simulink model "sensor"  (Simulink 4.00)
settings: Solver=ode45  StartTime=0.0  StopTime=0.5  MaxStep=1/80000  RelTol=1e-3
settings Model: LastModifiedBy=Gui

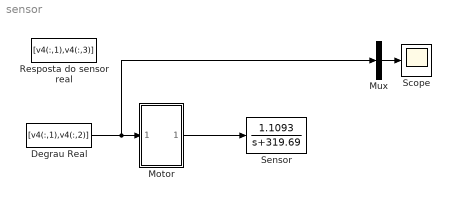
== system sensor ==
  Degrau Real : FromWorkspace  VariableName=[v4(:,1),v4(:,2)]  SampleTime=0  OutputAfterFinalValue=Extrapolation
  Motor : Subsystem
      settings: RTWFcnNameOpts=Auto  RTWFileNameOpts=Auto
  Mux : Mux  Inputs=3
  Resposta do sensor real : FromWorkspace  VariableName=[v4(:,1),v4(:,3)]  SampleTime=0  OutputAfterFinalValue=Extrapolation
  Scope : Scope
      settings: TimeRange=0.5  YMin=0  YMax=10  SaveToWorkspace=off  SaveName=ScopeData  MaxDataPoints=5000
  "Sensor " : TransferFcn  Numerator=1.1093  Denominator=[1 319.69]  AbsoluteTolerance=auto  Realization=auto
  wires:
  Degrau Real/1 -> Motor/1(In1), Mux/2
  Mux/1 -> Scope/1
  Motor/1(Out1) -> "Sensor "/1

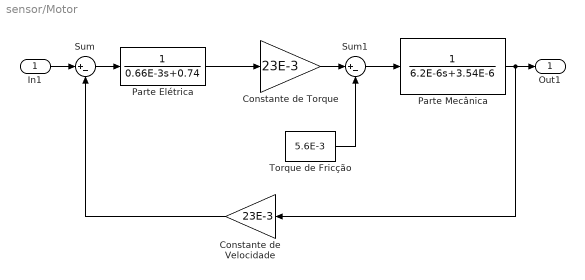
== system sensor/Motor ==
  In1 : Inport  Port=1  LatchInput=off
  Constante de Torque : Gain  Gain=23E-3  Multiplication=Element-wise(K.*u)  SaturateOnIntegerOverflow=on
  Constante de Velocidade : Gain  Orientation=left  Gain=23E-3  Multiplication=Element-wise(K.*u)  SaturateOnIntegerOverflow=on
  Parte Elétrica : TransferFcn  Numerator=[1]  Denominator=[0.66E-3 0.74]  AbsoluteTolerance=auto  Realization=auto
  Parte Mecânica : TransferFcn  Numerator=[1]  Denominator=[6.2E-6 3.54E-6]  AbsoluteTolerance=auto  Realization=auto
  Sum : Sum  Inputs=|+-  SaturateOnIntegerOverflow=on
  Sum1 : Sum  Inputs=|+-  SaturateOnIntegerOverflow=on
  Torque de Fricção : Constant  Value=5.6E-3
  Out1 : Outport  Port=1
  wires:
  Sum/1 -> Parte Elétrica/1
  Parte Elétrica/1 -> Constante de Torque/1
  Parte Mecânica/1 -> Constante de Velocidade/1, Out1/1
  Constante de Velocidade/1 -> Sum/2
  Constante de Torque/1 -> Sum1/1
  Sum1/1 -> Parte Mecânica/1
  Torque de Fricção/1 -> Sum1/2
  In1/1 -> Sum/1
